simulink model "discrete_complete_model"  (R2023b)
settings: Solver=VariableStepAuto  StartTime=0.0  StopTime=100  FixedStep=1e-3  RelTol=1e-3
values from neighbouring files (symbols this model uses):
  dt = time(i) - time(i-1)    [animation.m]
undefined symbols (not defined in the file or in its folder): adcs_ape_rad, adcs_noise_power, adcs_sample_time, d_distub2, d_disturb1, DiscIntNeverNeededParam, disturb_const, disturb_force1, disturb_force2, end_step1, end_step2, end_step3, end_time, end_value, gyro_noise_power, gyro_sample_time, gyro_walk_power, h_rw0, I_rw, I_sat, I_sat_inv, ini_step1, ini_step2, ini_step3, ini_value, K_daw, K_dI, K_domega, K_dq, motor_mask, omega0, Q_noise, quat0, R_noise, rw_noise_power, rw_sample_time, start_time, t_disturb1, t_disturb2, t_step1, t_step2, t_step3, tau_motor
libraries: sharedtransform x6, simulink x4, aerolibutil x3, sharedutil x3, simulink_extras x3, matrix_library x2, dspstat3 x2, eeGeneralControl x1
settings Model: Creator=Nahuel  LastModifiedBy=Nahuel

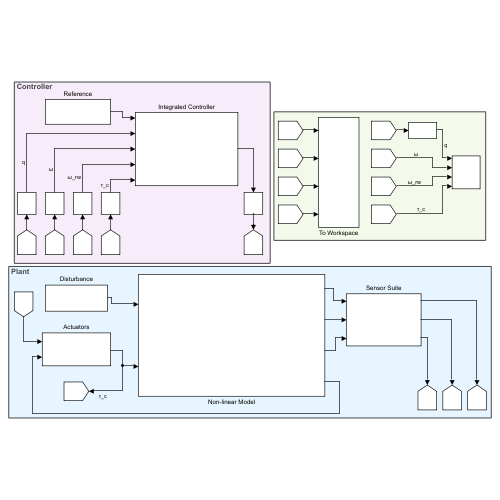
[thumbnail: Simulink's stored preview of the top-level diagram]
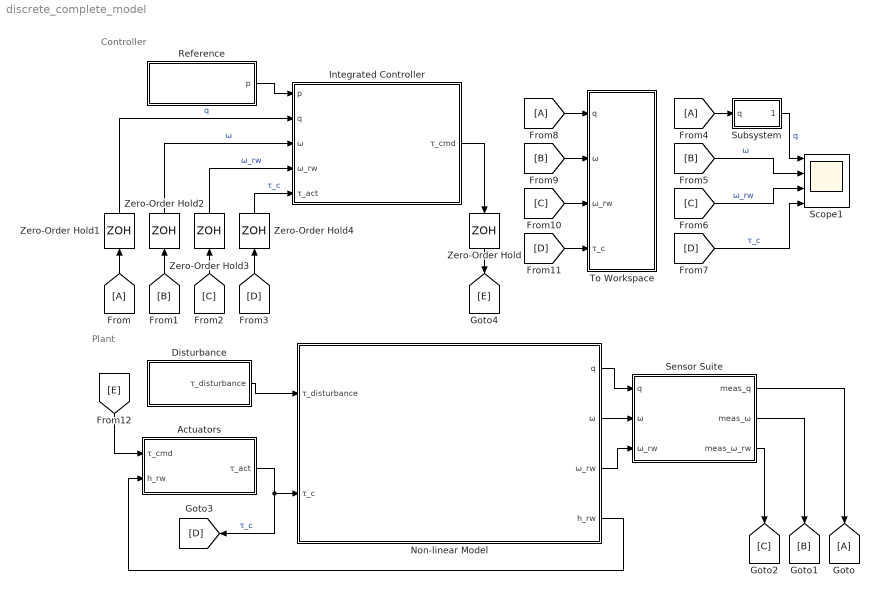
== system discrete_complete_model ==
  note: Controller
  note: Plant
  Actuators : Subsystem
  Disturbance : Subsystem
  From : From
  From4 : From
  From8 : From
  Goto : Goto
  Integrated Controller : Subsystem  TreatAsAtomicUnit=on  SystemSampleTime=dt
  Non-linear Model : Subsystem
  Reference : Subsystem
  Scope1 : Scope  NumInputPorts=4
  Sensor Suite : Subsystem  SystemSampleTime=0.001
  Subsystem : Subsystem
  To Workspace : Subsystem
  Zero-Order Hold{,1..4} (5 alike) : ZeroOrderHold  SampleTime=dt
  wires:
  Non-linear Model/3(ω_rw) -> Sensor Suite/3(ω_rw)
  Non-linear Model/2(ω) -> Sensor Suite/2(ω)
  Non-linear Model/1(q) -> Sensor Suite/1(q)
  Zero-Order Hold1/1 -> Integrated Controller/2(q)  "q"
  Zero-Order Hold2/1 -> Integrated Controller/3(ω)  "ω"
  Zero-Order Hold3/1 -> Integrated Controller/4(ω_rw)  "ω_rw"
  Disturbance/1(τ_disturbance) -> Non-linear Model/1(τ_disturbance)
  Non-linear Model/4(h_rw) -> Actuators/2(h_rw)
  Integrated Controller/1(τ_cmd) -> Zero-Order Hold/1
  Reference/1(p) -> Integrated Controller/1(p)
  Actuators/1(τ_act) -> Non-linear Model/2(τ_c), [D]  "τ_c"
  Sensor Suite/1(meas_q) -> Goto/1
  Zero-Order Hold4/1 -> Integrated Controller/5(τ_act)  "τ_c"
  Sensor Suite/2(meas_ω) -> [B]
  [B] -> Zero-Order Hold2/1
  Sensor Suite/3(meas_ω_rw) -> [C]
  [C] -> Zero-Order Hold3/1
  [D] -> Zero-Order Hold4/1
  [B] -> Scope1/2  "ω"
  [C] -> Scope1/3  "ω_rw"
  [D] -> Scope1/4  "τ_c"
  From8/1 -> To Workspace/1(q)
  [B] -> To Workspace/2(ω)
  [C] -> To Workspace/3(ω_rw)
  [D] -> To Workspace/4(τ_c)
  [E] -> Actuators/1(τ_cmd)
  Zero-Order Hold/1 -> [E]
  From/1 -> Zero-Order Hold1/1
  From4/1 -> Subsystem/1(q)
  Subsystem/1(angles) -> Scope1/1  "q"

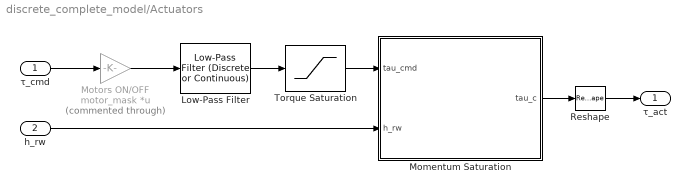
== system discrete_complete_model/Actuators ==
  τ_cmd : Inport
  h_rw : Inport  Port=2
  " Motors ON/OFF" : Gain  Commented=through  Gain=motor_mask  Multiplication=Matrix(K*u)
  Low-Pass Filter : eeGeneralControl/Low-Pass Filter (Discrete or Continuous)  K=1  T=tau_motor  B=inf  A=-inf  init_option=Inherited from block input  x0=0  Ts=0
  Momentum Saturation : MATLAB Function  TreatAsAtomicUnit=on
  Reshape : Reshape
  Torque Saturation : Saturate  UpperLimit=0.0002  LowerLimit=-0.0002
  τ_act : Outport
  wires:
  Torque Saturation/1 -> Momentum Saturation/1(tau_cmd)
  h_rw/1 -> Momentum Saturation/2(h_rw)
  Reshape/1 -> τ_act/1
  τ_cmd/1 -> " Motors ON/OFF"/1
  Momentum Saturation/1(tau_c) -> Reshape/1
  Low-Pass Filter/1 -> Torque Saturation/1
  " Motors ON/OFF"/1 -> Low-Pass Filter/1

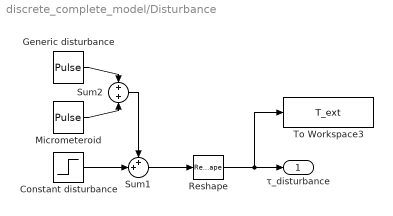
== system discrete_complete_model/Disturbance ==
  " Constant disturbance" : Step  Time=0  Before=[0, 0, 0]  After=disturb_const  SampleTime=0
  " Micrometeroid" : DiscretePulseGenerator  PulseType=Time based  Amplitude=disturb_force1  Period=300  PulseWidth=d_disturb1  PhaseDelay=t_disturb1
  Generic disturbance : DiscretePulseGenerator  PulseType=Time based  Amplitude=disturb_force2  Period=100  PulseWidth=d_distub2  PhaseDelay=t_disturb2
  Reshape : Reshape
  Sum1 : Sum  Inputs=++|
  Sum2 : Sum
  To Workspace3 : ToWorkspace  VariableName=T_ext  SaveFormat=Timeseries  SampleTime=-1
  τ_disturbance : Outport
  wires:
  " Constant disturbance"/1 -> Sum1/2
  " Micrometeroid"/1 -> Sum2/2
  Generic disturbance/1 -> Sum2/1
  Reshape/1 -> τ_disturbance/1, To Workspace3/1
  Sum1/1 -> Reshape/1
  Sum2/1 -> Sum1/1

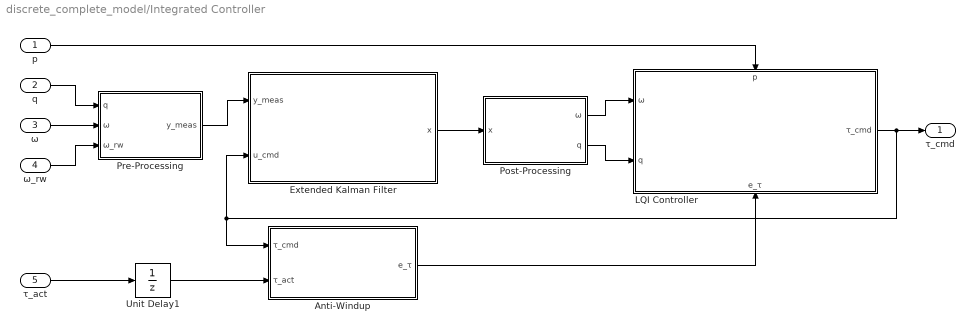
== system discrete_complete_model/Integrated Controller ==
  p : Inport
  q : Inport  Port=2
  ω : Inport  Port=3
  ω_rw : Inport  Port=4
  τ_act : Inport  Port=5
  Anti-Windup : Subsystem
  Extended Kalman Filter : Subsystem
  LQI Controller : Subsystem
      settings: PortSchema="{\"entries\":[{\"content\":{\"sides\":[{\"content\":{\"connectorIds\":[\"In1\",\"In2\"]},\"type\":\"ConnectorPlacement.EquallySpacedRectSide\",\"uuid\":\"2ebfe950-d43d-47a2-a975-d9ee473367e9\"},{\"content\":{\"connectorIds\":[\"Out1\"],\"side\":\"RIGHT\"},\"type\":\"ConnectorPlacement.EquallySpacedRectSide\",\"uuid\":\"47fee382-8d93-4b13-ac31-5bc139d18ea2\"},{\"content\":{\"connectorIds\":[\"In3\"],\"side\":\"TOP\"},\"type\":\"ConnectorPlacement.EquallySpacedRectSide\",\"uuid\":\"edc24e11-9160-40c2-ad00-b723775598ab\"},{\"content\":{\"connectorIds\":[\"In4\"],\"side\":\"BOTTOM\"},\"type\":\"ConnectorPlacement.EquallySpacedRectSide\",\"uuid\":\"72f7bbeb-14cb-4018-a4a4-cb6cc2af2049\"}]},\"type\":\"ConnectorPlacement.EquallySpacedConnector\",\"uuid\":\"b3cd18a8-1b82-4223-b3fb-1fd10c00f843\"}],\"packageUris\":[\"http://schema.mathworks.com/mf0/Connector/R2020b\"],\"version\":\"1.0\"}"
  Post-Processing : Subsystem
  Pre-Processing : Subsystem
  Unit Delay1 : UnitDelay  SampleTime=-1  HasFrameUpgradeWarning=on
  τ_cmd : Outport
  wires:
  ω/1 -> Pre-Processing/2(ω)
  Post-Processing/1(ω) -> LQI Controller/1(ω)
  Extended Kalman Filter/1(x) -> Post-Processing/1(x)
  Post-Processing/2(q) -> LQI Controller/2(q)
  Pre-Processing/1(y_meas) -> Extended Kalman Filter/1(y_meas)
  p/1 -> LQI Controller/3(p)
  q/1 -> Pre-Processing/1(q)
  ω_rw/1 -> Pre-Processing/3(ω_rw)
  τ_act/1 -> Unit Delay1/1
  Anti-Windup/1(e_τ) -> LQI Controller/4(e_τ)
  Unit Delay1/1 -> Anti-Windup/2(τ_act)
  LQI Controller/1(τ_cmd) -> τ_cmd/1, Anti-Windup/1(τ_cmd), Extended Kalman Filter/2(u_cmd)

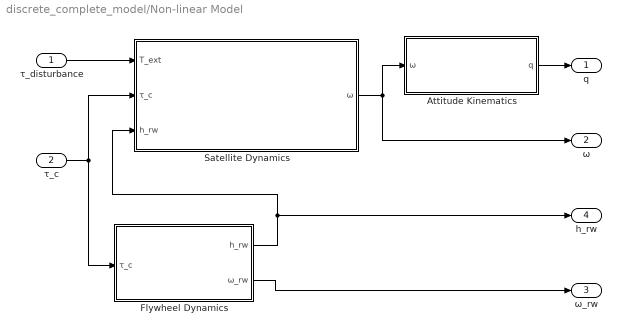
== system discrete_complete_model/Non-linear Model ==
  τ_disturbance : Inport
  τ_c : Inport  Port=2
  Attitude Kinematics : Subsystem
  Flywheel Dynamics : Subsystem
  Satellite Dynamics : Subsystem
  q : Outport
  ω : Outport  Port=2
  ω_rw : Outport  Port=3
  h_rw : Outport  Port=4
  wires:
  Flywheel Dynamics/1(h_rw) -> Satellite Dynamics/3(h_rw), h_rw/1
  Satellite Dynamics/1(ω) -> ω/1, Attitude Kinematics/1(ω)
  τ_c/1 -> Flywheel Dynamics/1(τ_c), Satellite Dynamics/2(τ_c)
  τ_disturbance/1 -> Satellite Dynamics/1(T_ext)
  Flywheel Dynamics/2(ω_rw) -> ω_rw/1
  Attitude Kinematics/1(q) -> q/1

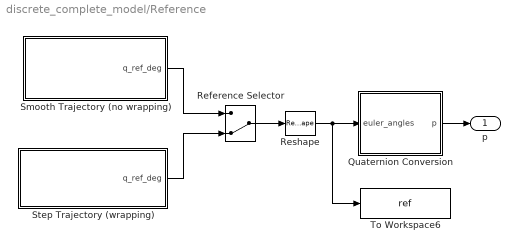
== system discrete_complete_model/Reference ==
  Quaternion Conversion : Subsystem
  Reference Selector : ManualSwitch  CurrentSetting=0
  Reshape : Reshape
  Smooth Trajectory (no wrapping) : Subsystem
  Step Trajectory (wrapping) : Subsystem
  To Workspace6 : ToWorkspace  VariableName=ref  SaveFormat=Timeseries  SampleTime=-1
  p : Outport
  wires:
  Reference Selector/1 -> Reshape/1
  Quaternion Conversion/1(p) -> p/1
  Reshape/1 -> Quaternion Conversion/1(euler_angles), To Workspace6/1
  Smooth Trajectory (no wrapping)/1(q_ref_deg) -> Reference Selector/1
  Step Trajectory (wrapping)/1(q_ref_deg) -> Reference Selector/2

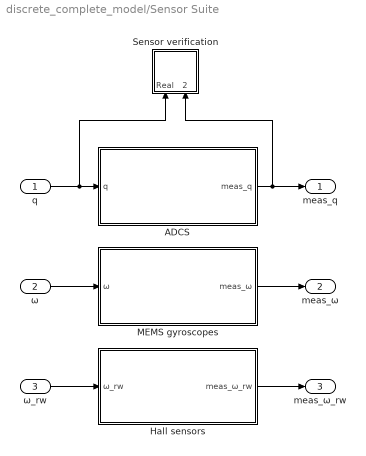
== system discrete_complete_model/Sensor Suite ==
  q : Inport
  ω : Inport  Port=2
  ω_rw : Inport  Port=3
  ADCS : Subsystem
  Hall sensors : Subsystem
  MEMS gyroscopes : Subsystem
  Sensor verification : Subsystem
  meas_q : Outport
  meas_ω : Outport  Port=2
  meas_ω_rw : Outport  Port=3
  wires:
  ω_rw/1 -> Hall sensors/1(ω_rw)
  ω/1 -> MEMS gyroscopes/1(ω)
  Hall sensors/1(meas_ω_rw) -> meas_ω_rw/1
  q/1 -> ADCS/1(q), Sensor verification/1(Real)
  MEMS gyroscopes/1(meas_ω) -> meas_ω/1
  ADCS/1(meas_q) -> Sensor verification/2(Meas), meas_q/1

== system discrete_complete_model/Subsystem ==
  q : Inport
  Quaternions to Rotation Angles : sharedtransform/Quaternions to Rotation Angles  rotationOrder=ZYX  aMode=aMode
  Radians to Degrees : simulink_extras/Transformations/Radians to Degrees
  angles : Outport
  wires:
  Quaternions to Rotation Angles/1 -> Radians to Degrees/1
  q/1 -> Quaternions to Rotation Angles/1
  Radians to Degrees/1 -> angles/1

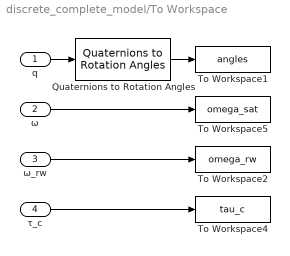
== system discrete_complete_model/To Workspace ==
  q : Inport
  ω : Inport  Port=2
  ω_rw : Inport  Port=3
  τ_c : Inport  Port=4
  Quaternions to Rotation Angles : sharedtransform/Quaternions to Rotation Angles  rotationOrder=ZYX  aMode=aMode
  To Workspace1 : ToWorkspace  VariableName=angles  SaveFormat=Timeseries  SampleTime=-1
  To Workspace2 : ToWorkspace  VariableName=omega_rw  SaveFormat=Timeseries  SampleTime=-1
  To Workspace4 : ToWorkspace  VariableName=tau_c  SaveFormat=Timeseries  SampleTime=-1
  To Workspace5 : ToWorkspace  VariableName=omega_sat  SaveFormat=Timeseries  SampleTime=-1
  wires:
  ω_rw/1 -> To Workspace2/1
  ω/1 -> To Workspace5/1
  τ_c/1 -> To Workspace4/1
  q/1 -> Quaternions to Rotation Angles/1
  Quaternions to Rotation Angles/1 -> To Workspace1/1

== system discrete_complete_model/Integrated Controller/Anti-Windup ==
  τ_cmd : Inport
  τ_act : Inport  Port=2
  Dead Zone : DeadZone  LowerValue=-0.001e-3  UpperValue=0.001e-3
  Gain : Gain  Gain=K_daw  Multiplication=Matrix(K*u)
  Sum : Sum  Inputs=+-
  e_τ : Outport
  wires:
  Sum/1 -> Dead Zone/1
  τ_act/1 -> Sum/2
  Gain/1 -> e_τ/1
  τ_cmd/1 -> Sum/1
  Dead Zone/1 -> Gain/1

== system discrete_complete_model/Integrated Controller/Extended Kalman Filter ==
  y_meas : Inport
  u_cmd : Inport  Port=2
  EKF step : MATLAB Function  TreatAsAtomicUnit=on
  Unit Delay : UnitDelay  InitialCondition=1e-3 * eye(10)  SampleTime=-1  HasFrameUpgradeWarning=on
  Unit Delay1 : UnitDelay  InitialCondition=[1;0;0;0; 0;0;0; 0;0;0]  SampleTime=-1  HasFrameUpgradeWarning=on
  Unit Delay2 : UnitDelay  InitialCondition=[0; 0; 0]  SampleTime=-1  HasFrameUpgradeWarning=on
  x : Outport
  wires:
  EKF step/2(P_next) -> Unit Delay/1
  Unit Delay1/1 -> EKF step/1(x_prev)
  EKF step/1(x_next) -> x/1, Unit Delay1/1
  Unit Delay/1 -> EKF step/2(P_prev)
  u_cmd/1 -> Unit Delay2/1
  y_meas/1 -> EKF step/4(y_meas)
  Unit Delay2/1 -> EKF step/3(u_cmd)

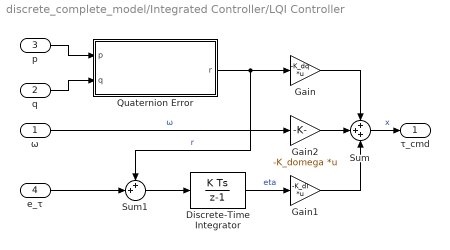
== system discrete_complete_model/Integrated Controller/LQI Controller ==
  ω : Inport
  q : Inport  Port=2
  p : Inport  Port=3
  e_τ : Inport  Port=4
  Discrete-Time Integrator : DiscreteIntegrator  InitialCondition=[0;0;0]  SampleTime=-1  UpperSaturationLimit=0.2e-3  LowerSaturationLimit=-0.2e-3  ICPrevOutput=DiscIntNeverNeededParam  ICPrevScaledInput=DiscIntNeverNeededParam
  Gain : Gain  Gain=-K_dq  Multiplication=Matrix(K*u)
  Gain1 : Gain  Gain=-K_dI  Multiplication=Matrix(K*u)
  Gain2 : Gain  Gain=-K_domega  Multiplication=Matrix(K*u)
  Quaternion Error : Subsystem
  Sum : Sum  Inputs=+++
  Sum1 : Sum  Inputs=++|
  τ_cmd : Outport
  wires:
  Discrete-Time Integrator/1 -> Gain1/1  "eta"
  Sum/1 -> τ_cmd/1  "x"
  ω/1 -> Gain2/1  "ω"
  Gain/1 -> Sum/1
  p/1 -> Quaternion Error/1(p)
  q/1 -> Quaternion Error/2(q)
  e_τ/1 -> Sum1/2
  Sum1/1 -> Discrete-Time Integrator/1
  Gain1/1 -> Sum/3
  Gain2/1 -> Sum/2
  Quaternion Error/1(r) -> Sum1/1, Gain/1  "r"

== system discrete_complete_model/Integrated Controller/Post-Processing ==
  x : Inport
  Selector : Selector  InputPortWidth=10  IndexOptions=Index vector (dialog)  Indices=[5 6 7]  OutputSizes=1
  Selector2 : Selector  InputPortWidth=10  IndexOptions=Index vector (dialog)  Indices=[1 2 3 4]  OutputSizes=1
  ω : Outport
  q : Outport  Port=2
  wires:
  x/1 -> Selector/1, Selector2/1
  Selector/1 -> ω/1
  Selector2/1 -> q/1

== system discrete_complete_model/Integrated Controller/Pre-Processing ==
  q : Inport
  ω : Inport  Port=2
  ω_rw : Inport  Port=3
  Gain : Gain  Gain=I_rw
  Mux : Mux  Inputs=3
  Quaternion Normalize : sharedutil/Quaternion Normalize  aMode=aMode
  y_meas : Outport
  wires:
  Mux/1 -> y_meas/1
  ω_rw/1 -> Gain/1
  ω/1 -> Mux/2  "ω"
  Gain/1 -> Mux/3  "h_rw"
  q/1 -> Quaternion Normalize/1
  Quaternion Normalize/1 -> Mux/1  "q"

== system discrete_complete_model/Non-linear Model/Attitude Kinematics ==
  ω : Inport
  Integrator : Integrator  InitialCondition=quat0
  Quaternion Normalize : sharedutil/Quaternion Normalize  aMode=aMode
  Ω Function : MATLAB Function  TreatAsAtomicUnit=on
  q : Outport
  wires:
  Integrator/1 -> Quaternion Normalize/1  "q"
  Quaternion Normalize/1 -> Ω Function/2(q), q/1  "q"
  Ω Function/1(q_dot) -> Integrator/1  "dot_q"
  ω/1 -> Ω Function/1(omega)

== system discrete_complete_model/Non-linear Model/Flywheel Dynamics ==
  τ_c : Inport
  Gain : Gain  Gain=-1
  Gain1 : Gain  Gain=1/I_rw
  Integrator2 : Integrator  InitialCondition=h_rw0
  h_rw : Outport
  ω_rw : Outport  Port=2
  wires:
  Integrator2/1 -> h_rw/1, Gain1/1  "h_rw"
  Gain/1 -> Integrator2/1  "dot_h_rw"
  τ_c/1 -> Gain/1
  Gain1/1 -> ω_rw/1

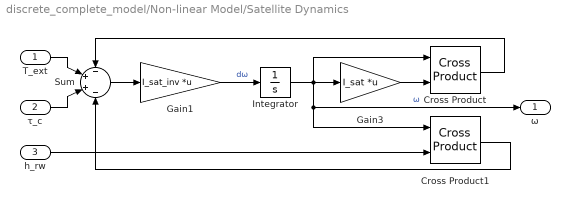
== system discrete_complete_model/Non-linear Model/Satellite Dynamics ==
  T_ext : Inport
  τ_c : Inport  Port=2
  h_rw : Inport  Port=3
  Cross Product : matrix_library/Cross Product
  Cross Product1 : matrix_library/Cross Product
  Gain1 : Gain  Gain=I_sat_inv  Multiplication=Matrix(K*u)
  Gain3 : Gain  Gain=I_sat  Multiplication=Matrix(K*u)
  Integrator : Integrator  InitialCondition=omega0
  Sum : Sum  Inputs=-++-
  ω : Outport
  wires:
  Gain1/1 -> Integrator/1  "dω​"
  Integrator/1 -> Cross Product1/1, ω/1, Cross Product/1, Gain3/1  "ω"
  Sum/1 -> Gain1/1
  T_ext/1 -> Sum/2
  τ_c/1 -> Sum/3
  Gain3/1 -> Cross Product/2
  h_rw/1 -> Cross Product1/2
  Cross Product/1 -> Sum/1
  Cross Product1/1 -> Sum/4

== system discrete_complete_model/Reference/Quaternion Conversion ==
  euler_angles : Inport
  Degrees to Radians : simulink_extras/Transformations/Degrees to Radians
  Quaternion Normalize : sharedutil/Quaternion Normalize  aMode=aMode
  Rotation Angles to Quaternions : sharedtransform/Rotation Angles to Quaternions  rotationOrder=ZYX  aMode=aMode
  XYZ : Demux  Outputs=3
  ZYX : Mux  Inputs=3
  p : Outport
  wires:
  XYZ/3 -> ZYX/1
  XYZ/1 -> ZYX/3
  Degrees to Radians/1 -> XYZ/1
  Quaternion Normalize/1 -> p/1
  XYZ/2 -> ZYX/2
  ZYX/1 -> Rotation Angles to Quaternions/1
  euler_angles/1 -> Degrees to Radians/1
  Rotation Angles to Quaternions/1 -> Quaternion Normalize/1

== system discrete_complete_model/Reference/Smooth Trajectory (no wrapping) ==
  Clock : Clock
  Constant : Constant  Value=start_time
  Constant1 : Constant  Value=end_time
  Constant2 : Constant  Value=ini_value
  Constant3 : Constant  Value=end_value
  MATLAB Function : MATLAB Function  TreatAsAtomicUnit=on
  q_ref_deg : Outport
  wires:
  Constant2/1 -> MATLAB Function/4(start_deg_vec)
  Constant1/1 -> MATLAB Function/3(duration_s)
  Constant/1 -> MATLAB Function/2(t_start)
  Clock/1 -> MATLAB Function/1(t)
  MATLAB Function/1(q_ref_deg) -> q_ref_deg/1
  Constant3/1 -> MATLAB Function/5(end_deg_vec)

== system discrete_complete_model/Reference/Step Trajectory (wrapping) ==
  Ref 1(°) : Step  Time=t_step1  Before=ini_step1  After=end_step1  SampleTime=0
  Ref 2(°) : Step  Time=t_step2  Before=ini_step2  After=end_step2  SampleTime=0
  Ref 3(°) : Step  Time=t_step3  Before=ini_step3  After=end_step3  SampleTime=0
  Sum : Sum  Inputs=+++
  q_ref_deg : Outport
  wires:
  Ref 1(°)/1 -> Sum/1
  Ref 2(°)/1 -> Sum/2
  Sum/1 -> q_ref_deg/1
  Ref 3(°)/1 -> Sum/3

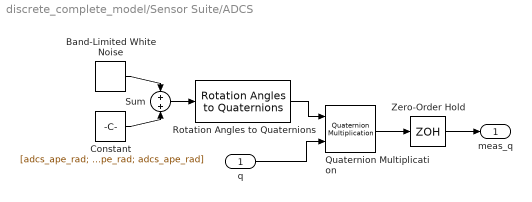
== system discrete_complete_model/Sensor Suite/ADCS ==
  q : Inport
  Band-Limited White Noise : simulink/Sources/Band-Limited White Noise  Cov=[adcs_noise_power, adcs_noise_power, adcs_noise_power]  Ts=adcs_sample_time  seed=[23341, 42342, 53453]
  Constant : Constant  Value=[adcs_ape_rad; adcs_ape_rad; adcs_ape_rad]
  Quaternion Multiplication : aerolibutil/Quaternion Multiplication
  Rotation Angles to Quaternions : sharedtransform/Rotation Angles to Quaternions  rotationOrder=ZYX  aMode=aMode
  Sum : Sum
  Zero-Order Hold : ZeroOrderHold  SampleTime=adcs_sample_time
  meas_q : Outport
  wires:
  q/1 -> Quaternion Multiplication/2
  Band-Limited White Noise/1 -> Sum/1
  Sum/1 -> Rotation Angles to Quaternions/1
  Constant/1 -> Sum/2
  Rotation Angles to Quaternions/1 -> Quaternion Multiplication/1
  Zero-Order Hold/1 -> meas_q/1
  Quaternion Multiplication/1 -> Zero-Order Hold/1

== system discrete_complete_model/Sensor Suite/Hall sensors ==
  ω_rw : Inport
  Band-Limited White Noise : simulink/Sources/Band-Limited White Noise  Cov=[rw_noise_power, rw_noise_power, rw_noise_power]  Ts=rw_sample_time  seed=[99, 88, 77]
  Quantizer : Quantizer  QuantizationInterval=rw_quantization_interval
  Sum : Sum  Inputs=|++
  Zero-Order Hold : ZeroOrderHold  SampleTime=rw_sample_time
  meas_ω_rw : Outport
  wires:
  ω_rw/1 -> Sum/1
  Zero-Order Hold/1 -> meas_ω_rw/1
  Band-Limited White Noise/1 -> Sum/2
  Sum/1 -> Quantizer/1
  Quantizer/1 -> Zero-Order Hold/1

== system discrete_complete_model/Sensor Suite/MEMS gyroscopes ==
  ω : Inport
  Band-Limited White Noise : simulink/Sources/Band-Limited White Noise  Cov=[gyro_noise_power, gyro_noise_power, gyro_noise_power]  Ts=gyro_sample_time  seed=[12, 34, 56]
      link override White Noise: SampleTime=Ts
  Band-Limited White Noise1 : simulink/Sources/Band-Limited White Noise  Cov=[gyro_walk_power, gyro_walk_power, gyro_walk_power]  Ts=gyro_sample_time  seed=[15, 39, 63]
      link override White Noise: SampleTime=Ts
  Integrator : Integrator  InitialCondition=[0, 0, 0]
  Sum : Sum  Inputs=+++
  Zero-Order Hold : ZeroOrderHold  SampleTime=gyro_sample_time
  meas_ω : Outport
  wires:
  ω/1 -> Sum/2
  Band-Limited White Noise1/1 -> Integrator/1
  Band-Limited White Noise/1 -> Sum/1
  Zero-Order Hold/1 -> meas_ω/1
  Sum/1 -> Zero-Order Hold/1
  Integrator/1 -> Sum/3

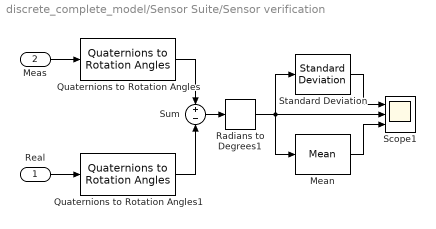
== system discrete_complete_model/Sensor Suite/Sensor verification ==
  Real : Inport
  Meas : Inport  Port=2
  Mean : dspstat3/Mean  run=off  InputProcessing=Columns as channels (frame based)  reset_popup=None  directionMode=Entire input  dimension=1  roiEnable=off  roiType=Rectangles  roiPortion=Entire ROI  roiOutput=Individual statistics for each ROI  roiFlag=off  roundingMode=Floor  overflowMode=off  outputDataTypeStr=Inherit: Same as accumulator  outputMin=[]  outputMax=[]  outputLastDataTypeStr=Inherit: Same as accumulator
  Quaternions to Rotation Angles : sharedtransform/Quaternions to Rotation Angles  rotationOrder=ZYX  aMode=aMode
  Quaternions to Rotation Angles1 : sharedtransform/Quaternions to Rotation Angles  rotationOrder=ZYX  aMode=aMode
  Radians to Degrees1 : simulink_extras/Transformations/Radians to Degrees
  Scope1 : Scope  NumInputPorts=3
  Standard Deviation : dspstat3/Standard Deviation  run=off  directionMode=Each column  dimension=1  InputProcessing=Columns as channels (frame based)  reset_popup=None  roiEnable=off  roiType=Rectangles  roiPortion=Entire ROI  roiOutput=Individual statistics for each ROI  roiFlag=off
  Sum : Sum  Inputs=+-
  wires:
  Sum/1 -> Radians to Degrees1/1
  Meas/1 -> Quaternions to Rotation Angles/1
  Standard Deviation/1 -> Scope1/1
  Mean/1 -> Scope1/3
  Real/1 -> Quaternions to Rotation Angles1/1
  Quaternions to Rotation Angles/1 -> Sum/1
  Quaternions to Rotation Angles1/1 -> Sum/2
  Radians to Degrees1/1 -> Mean/1, Scope1/2, Standard Deviation/1

== system discrete_complete_model/Integrated Controller/LQI Controller/Quaternion Error ==
  p : Inport
  q : Inport  Port=2
  Quaternion Conjugate : aerolibutil/Quaternion Conjugate
  Quaternion Multiplication : aerolibutil/Quaternion Multiplication
  Selector : Selector  InputPortWidth=4  IndexOptions=Index vector (dialog)  Indices=[2 3 4]  OutputSizes=1
  Shortest Path : Subsystem
  r : Outport
  wires:
  p/1 -> Quaternion Conjugate/1
  Quaternion Multiplication/1 -> Selector/1, Shortest Path/2(r0)
  Quaternion Conjugate/1 -> Quaternion Multiplication/1  "p*"
  q/1 -> Quaternion Multiplication/2  "q"
  Selector/1 -> Shortest Path/1(rv)  "r"
  Shortest Path/1(r_short) -> r/1

== system discrete_complete_model/Integrated Controller/LQI Controller/Quaternion Error/Shortest Path ==
  rv : Inport
  r0 : Inport  Port=2
  Product : Product
  Selector1 : Selector  InputPortWidth=4  IndexOptions=Index vector (dialog)  Indices=[1]  OutputSizes=1
  Sign : Signum
  r_short : Outport
  wires:
  Product/1 -> r_short/1
  r0/1 -> Selector1/1
  Selector1/1 -> Sign/1
  Sign/1 -> Product/2
  rv/1 -> Product/1

== matlab function discrete_complete_model/Non-linear Model/Attitude Kinematics/Ω Function ==
  data: omega input; q_dot output; q input
function q_dot = fcn(omega, q)
    % omega is [3x1] vector (rad/s)
    % q is [4x1] quaternion vector
    
    wx = omega(1);
    wy = omega(2);
    wz = omega(3);
    
    % The Skew-Symmetric Matrix Omega
    Om = [ 0, -wx, -wy, -wz;
           wx,  0,   wz, -wy;
           wy, -wz,  0,   wx;
           wz,  wy, -wx,  0 ];
           
    % Calculate derivative
    q_dot = 1/2 * Om * q;
end

== matlab function discrete_complete_model/Actuators/Momentum Saturation ==
  data: tau_cmd input; tau_c output; h_rw input
function tau_c = saturation_logic(tau_cmd, h_rw)
    % Inputs are now 3x1 Vectors
    % Output is a 3x1 Vector
    
    h_limit = 0.0006; % 0.6 mNms
    
    % Initialize output
    tau_c = zeros(3,1);
    
    % Loop through each wheel
    for i = 1:3
        current_h = h_rw(i);
        current_tau = tau_cmd(i);
        
        % Logic: If full AND trying to push further, cut torque
        % Remember: tau_cmd < 0 means acceleration (positive h_dot)
        if (current_h >= h_limit) && (current_tau < 0)
            tau_c(i) = 0;
        elseif (current_h <= -h_limit) && (current_tau > 0)
            tau_c(i) = 0;
        else
            tau_c(i) = current_tau;
        end
    end
end

== matlab function discrete_complete_model/Integrated Controller/Extended Kalman Filter/EKF step ==
  data: x_prev input; x_next output; P_prev input; u_cmd input; y_meas input; P_next output; I_sat parameter; I_sat_inv parameter; dt parameter; R_noise parameter; Q_noise parameter
function [x_next, P_next] = ekf_step_discrete(x_prev, P_prev, u_cmd, y_meas, I_sat, I_sat_inv, dt, R_noise, Q_noise)
    % Performs one discrete time step of the Extended Kalman Filter.

    % 0. INPUT SATURATION MODEL
    MAX_TORQUE = 0.0002; % 0.2 mNm
    MAX_MOMENTUM = 0.0006; % 0.6 mNms
    
    % Clamp Torque Magnitude
    u_limited = max(min(u_cmd, MAX_TORQUE), -MAX_TORQUE);
    
    % Apply Momentum Speed Limit Logic
    h_est = x_prev(8:10); 
    u_act = zeros(3,1);
    
    for i = 1:3
        % Check if adding torque would exceed momentum limits
        if (h_est(i) >= MAX_MOMENTUM) && (u_limited(i) < 0)
            u_act(i) = 0; % Wheel is full, cannot accelerate
        elseif (h_est(i) <= -MAX_MOMENTUM) && (u_limited(i) > 0)
            u_act(i) = 0; % Wheel is full negative
        else
            u_act(i) = u_limited(i);
        end
    end

    % 1. PREDICT STEP
    % Predict state forward using non-linear dynamics 
    
    % Euler integration method (faster but less accurate)
    %x_dot_pred = ekf_state_transition(x_prev, u_act, I_sat, I_sat_inv);
    %x_pred_raw = x_prev + x_dot_pred * dt;
    
    % Heun's Method (Runge-Kutta 2) (slower but accurate)
    % Calculate initial slope (k1)
    k1 = ekf_state_transition(x_prev, u_act, I_sat, I_sat_inv);
    % Predict end state using Euler guess
    x_guess = x_prev + k1 * dt;
    % Calculate slope at the guess point (k2)
    k2 = ekf_state_transition(x_guess, u_act, I_sat, I_sat_inv);
    % Average slopes and take final step
    x_pred_raw = x_prev + (dt/2) * (k1 + k2);
    
    % Normalize Predicted Quaternion to prevent drift
    q_pred = x_pred_raw(1:4) / norm(x_pred_raw(1:4));
    x_pred = [q_pred; x_pred_raw(5:10)];
    
    % Calculate Jacobian at previous state for covariance prediction
    A_jac = calculate_jacobian(x_prev, I_sat);
    
    % Predict Covariance forward (Discrete Time Linearized Propagation)
    % F_k = I + A*dt approx for discrete transition matrix
    F_k = eye(10) + A_jac * dt;
    % Formula for propagating Gaussian uncertainty
    P_pred = F_k * P_prev * F_k' + Q_noise;
    
    % 2. UPDATE STEP
    % Measurement Matrix H is Identity (all states are measured directly)
    H = eye(10);
    
    % Calculate Measurement Residual
    y_pred = H * x_pred; % Expected measurement based on prediction
    residual = y_meas - y_pred; % Innovation (new information)
    
    % Calculate Kalman Gain (K)
    S = H * P_pred * H' + R_noise; % Innovation covariance
    K = P_pred * H' / S;           % Optimal gain
    
    % Update State Estimate
    x_next_raw = x_pred + K * residual;
    
    % Normalize updated quaternion again just to be safe
    q_next = x_next_raw(1:4) / norm(x_next_raw(1:4));
    x_next = [q_next; x_next_raw(5:10)];
    
    % Update Covariance Estimate
    % Using Joseph form for numerical stability: P = (I-KH)P(I-KH)' + KRK'
    I10 = eye(10);
    P_next = (I10 - K*H) * P_pred * (I10 - K*H)' + K*R_noise*K';
end

== matlab function discrete_complete_model/Reference/Smooth Trajectory (no wrapping)/MATLAB Function ==
  data: t input; q_ref_deg output; t_start input; duration_s input; start_deg_vec input; end_deg_vec input
function q_ref_deg  = smooth_trajectory_vec(t, t_start, duration_s, start_deg_vec, end_deg_vec)
% Outputs:
%   q_ref_rad: Target position (Radians)

    % Initialize outputs
    q_ref_deg = zeros(3,1);

    % 1. Before start (Static)
    if t <= t_start
        q_ref_deg = start_deg_vec;

    % 2. After end (Static)
    elseif t >= (t_start + duration_s)
        q_ref_deg = end_deg_vec;

    % 3. Quintic Trajectory
    else
        % Time variables
        t_run = t - t_start;
        T = duration_s;
        tau = t_run / T; % Normalized time (0 to 1)
        
        % Distance to travel
        dist_vec = end_deg_vec - start_deg_vec;

        % Position Math
        scaling_pos = (10 * tau^3) - (15 * tau^4) + (6 * tau^5);
        q_ref_deg = start_deg_vec + (dist_vec * scaling_pos);     
    end
end
